simulink model "VTOL_sim"  (R2016b)
settings: Solver=ode45  StartTime=0.0  StopTime=P.t_end  RelTol=1e-3  EnableMultiTasking=on
InitFcn:
  | addpath ./..
  | VTOL_param
  | VTOLParamHW7
undefined symbols (not defined in the file or in its folder): P, VTOL_animation
libraries: simulink x2
settings Model: Creator=beard  LastModifiedBy=beard
settings DataIOCC: LimitDataPoints=on  SaveFormat=Array  SignalLoggingSaveFormat=ModelDataLogs
settings OptimizationCC: ExpressionDepthLimit=2147483647  InitFltsAndDblsToZero=on  LifeSpan=inf
settings DebuggingCC: UnderspecifiedInitializationDetection=Classic  MergeDetectMultiDrivingBlocksExec=none  SolverPrmCheckMsg=warning  FcnCallInpInsideContextMsg=warning  StateNameClashWarn=warning  SFUnexpectedBacktrackingDiag=warning  SFNoUnconditionalDefaultTransitionDiag=warning  SFExecutionAtInitializationDiag=none
settings HardwareCC: ProdBitPerPointer=32  ProdBitPerSizeT=32  ProdBitPerPtrDiffT=32  ProdLargestAtomicFloat=None  ProdIntDivRoundTo=Undefined  ProdEndianess=Unspecified  ProdWordSize=32  ProdHWDeviceType=32-bit Generic
settings ModelReferenceCC: PropagateSignalLabelsOutOfModel=off
settings GRTTargetCC: TargetLangStandard=C89/C90 (ANSI)  GeneratePreprocessorConditionals=Disable all  CombineOutputUpdateFcns=off  GRTInterface=on
settings ConfigComp: CovMetricSettings=dw  CovHtmlReporting=on  CovSaveCumulativeToWorkspaceVar=on  CovSaveSingleToWorkspaceVar=on  CovExternalEMLEnable=off

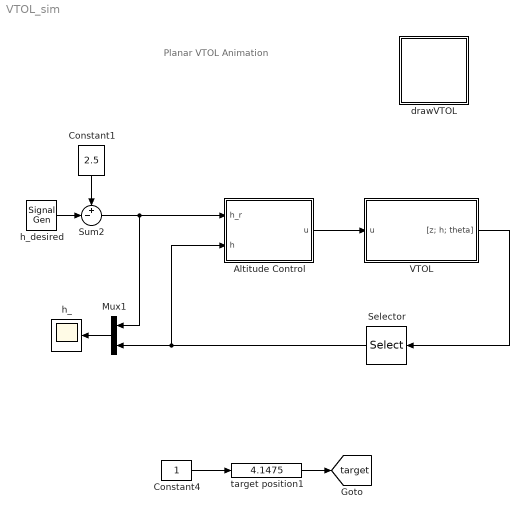
== system VTOL_sim ==
  note: Planar VTOL Animation
  Altitude Control : Subsystem
  Constant1 : Constant  Value=2.5
  Constant4 : Constant
  Mux1 : Mux  Inputs=2
  Selector : Selector  InputPortWidth=3  IndexOptions=Index vector (dialog)  Indices=[2]  OutputSizes=1
  Sum2 : Sum  Inputs=+-|
  VTOL : Subsystem
  drawVTOL : Subsystem
      mask Display: image(imread('tv.jpg'))
  h_ : Scope
  h_desired : SignalGenerator  WaveForm=square  Amplitude=2.5  Frequency=.01666666666
  target position1 : simulink/Math Operations/Slider Gain  low=0  gain=4.1475  high=6
  tag scope: target=global
  wires:
  VTOL/1("[z; h; theta]") -> Selector/1
  Mux1/1 -> h_/1
  Selector/1 -> Altitude Control/2(h), Mux1/2
  h_desired/1 -> Sum2/2
  Sum2/1 -> Mux1/1, Altitude Control/1(h_r)
  Constant1/1 -> Sum2/1
  Constant4/1 -> target position1/1
  target position1/1 -> [target]
  Altitude Control/1(u) -> VTOL/1(u)

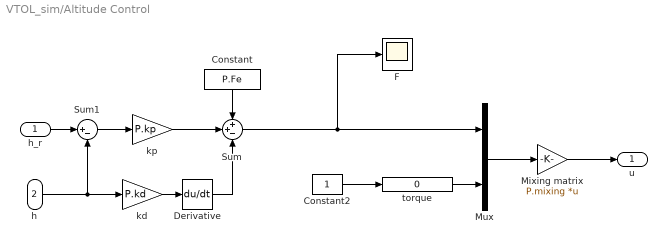
== system VTOL_sim/Altitude Control ==
  h_r : Inport
  h : Inport  Port=2
  Constant : Constant  Value=P.Fe
  Constant2 : Constant
  Derivative : Derivative
  F : Scope
  Mixing matrix : Gain  Gain=P.mixing  Multiplication=Matrix(K*u)
  Mux : Mux  Inputs=2
  Sum : Sum  Inputs=++-
  Sum1 : Sum  Inputs=|+-
  kd : Gain  Gain=P.kd
  kp : Gain  Gain=P.kp
  torque : simulink/Math Operations/Slider Gain  low=-1  gain=0  high=1
  u : Outport
  wires:
  Mixing matrix/1 -> u/1
  Sum/1 -> Mux/1, F/1
  kp/1 -> Sum/2
  h_r/1 -> Sum1/1
  Derivative/1 -> Sum/3
  Sum1/1 -> kp/1
  Constant/1 -> Sum/1
  h/1 -> kd/1, Sum1/2
  torque/1 -> Mux/2
  Mux/1 -> Mixing matrix/1
  kd/1 -> Derivative/1
  Constant2/1 -> torque/1

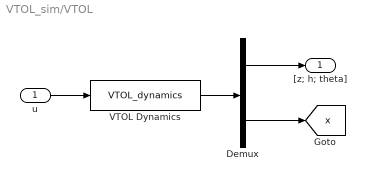
== system VTOL_sim/VTOL ==
  u : Inport
  Demux : Demux  Outputs=[3;6]
  VTOL Dynamics : S-Function  FunctionName=VTOL_dynamics  Parameters=P  SFunctionDeploymentMode=off  EnableBusSupport=off
  "[z; h; theta]" : Outport
  tag scope: x=global
  wires:
  Demux/2 -> [x]
  Demux/1 -> "[z; h; theta]"/1
  VTOL Dynamics/1 -> Demux/1
  u/1 -> VTOL Dynamics/1

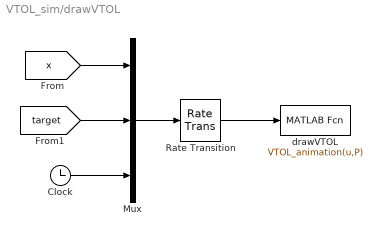
== system VTOL_sim/drawVTOL ==
  Clock : Clock
  Mux : Mux  Inputs=3
  Rate Transition : RateTransition  OutPortSampleTime=P.t_plot
  drawVTOL : MATLABFcn  MATLABFcn=VTOL_animation(u,P)  OutputDimensions=0
  wires:
  [target] -> Mux/2
  Rate Transition/1 -> drawVTOL/1
  Clock/1 -> Mux/3
  [x] -> Mux/1
  Mux/1 -> Rate Transition/1
